simulink model "MdXX_RspOutComm"  (R2018b)
settings: Solver=FixedStepDiscrete  StartTime=0.0  StopTime=10.0  FixedStep=0.01  RelTol=1e-3
undefined symbols (not defined in the file or in its folder): KeSMSuRspStatHldTm_Val
libraries: RspLib x60
(part 1 of 2)
settings Model: Creator=sn2xws  LastModifiedBy=sn2xws
settings DataIOCC: SaveFormat=StructureWithTime
settings OptimizationCC: DefaultParameterBehavior=Inlined  EnhancedBackFolding=on  PassReuseOutputArgsAs=Individual arguments  ZeroExternalMemoryAtStartup=off  ZeroInternalMemoryAtStartup=off  OptimizeBlockOrder=speed  DifferentSizesBufferReuse=on  OptimizationCustomize=off
settings DebuggingCC: ParameterTunabilityLossMsg=error
settings ModelReferenceCC: ModelReferenceNumInstancesAllowed=Single
settings SFSimCC: MATLABDynamicMemAlloc=off
settings RTWCC: SystemTargetFile=autosar.tlc  GenCodeOnly=on  TemplateMakefile=ert_default_tmf  Description=AUTOSAR  GenerateReport=on  IncludeHyperlinkInReport=on  LaunchReport=on  GenerateTraceInfo=on  GenerateTraceReport=on  GenerateTraceReportSl=on  GenerateTraceReportSf=on  GenerateTraceReportEml=on
settings CodeAppCC: ForceParamTrailComments=on  IgnoreCustomStorageClasses=off  OperatorAnnotations=on  SimulinkDataObjDesc=on  SFDataObjDesc=on  InsertBlockDesc=on
settings STFCustomTargetCC: TargetLangStandard=C99 (ISO)  MultiwordLength=256  ParMdlRefBuildCompliant=on  CompOptLevelCompliant=on  IncludeMdlTerminateFcn=off  CombineOutputUpdateFcns=on  SuppressErrorStatus=on  ERTCustomFileBanners=on  SupportNonFinite=off  SupportComplex=off  SupportContinuousTime=off  SupportNonInlinedSFcns=off  RemoveResetFunc=on  MATLABClassNameForMDSCustomization=Simulink.SoftwareTarget.ERTCustomization  AutosarCompliant=on  UseToolchainInfoCompliant=on  LookupTableObjectStructAxisOrder=2,1,3,4,...  LUTObjectStructOrderEvenSpacing=Size,Table,Breakpoints  SystemTargetFile=autosar.tlc
settings ERTTargetCC: TargetLangStandard=C99 (ISO)  ConcurrentExecutionCompliant=off  IncludeMdlTerminateFcn=off  SuppressErrorStatus=on  SupportNonFinite=off  SupportComplex=off  ModelStepFunctionPrototypeControlCompliant=off  CPPClassGenCompliant=off  AutosarCompliant=on  LookupTableObjectStructAxisOrder=2,1,3,4,...  LUTObjectStructOrderEvenSpacing=Size,Table,Breakpoints  InlinedParameterPlacement=NonHierarchical  ERTCustomFileTemplate=example_file_process.tlc

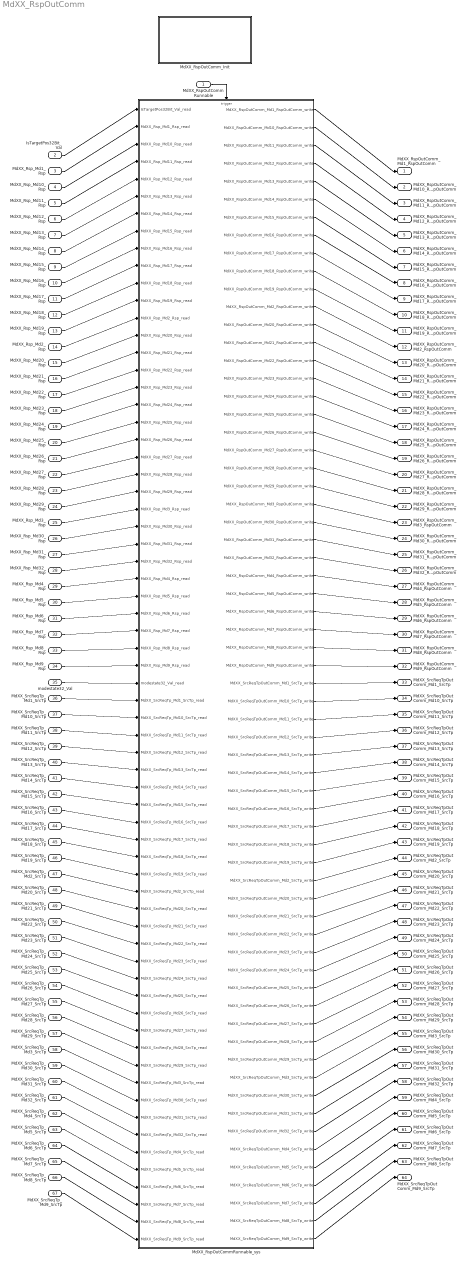
== system MdXX_RspOutComm ==
  MdXX_RspOutCommRunnable : Inport  SampleTime=0.01  OutputFunctionCall=on
  IsTargetPos32Bit_Val : Inport  Port=2  OutDataTypeStr=uint32  PortDimensions=1
  MdXX_Rsp_Md1_Rsp : Inport  Port=3  OutDataTypeStr=Enum: MdRspLocal2  PortDimensions=1
  MdXX_Rsp_Md10_Rsp : Inport  Port=4  OutDataTypeStr=Enum: MdRspLocal2  PortDimensions=1
  MdXX_Rsp_Md11_Rsp : Inport  Port=5  OutDataTypeStr=Enum: MdRspLocal2  PortDimensions=1
  MdXX_Rsp_Md12_Rsp : Inport  Port=6  OutDataTypeStr=Enum: MdRspLocal2  PortDimensions=1
  MdXX_Rsp_Md13_Rsp : Inport  Port=7  OutDataTypeStr=Enum: MdRspLocal2  PortDimensions=1
  MdXX_Rsp_Md14_Rsp : Inport  Port=8  OutDataTypeStr=Enum: MdRspLocal2  PortDimensions=1
  MdXX_Rsp_Md15_Rsp : Inport  Port=9  OutDataTypeStr=Enum: MdRspLocal2  PortDimensions=1
  MdXX_Rsp_Md16_Rsp : Inport  Port=10  OutDataTypeStr=Enum: MdRspLocal2  PortDimensions=1
  MdXX_Rsp_Md17_Rsp : Inport  Port=11  OutDataTypeStr=Enum: MdRspLocal2  PortDimensions=1
  MdXX_Rsp_Md18_Rsp : Inport  Port=12  OutDataTypeStr=Enum: MdRspLocal2  PortDimensions=1
  MdXX_Rsp_Md19_Rsp : Inport  Port=13  OutDataTypeStr=Enum: MdRspLocal2  PortDimensions=1
  MdXX_Rsp_Md2_Rsp : Inport  Port=14  OutDataTypeStr=Enum: MdRspLocal2  PortDimensions=1
  MdXX_Rsp_Md20_Rsp : Inport  Port=15  OutDataTypeStr=Enum: MdRspLocal2  PortDimensions=1
  MdXX_Rsp_Md21_Rsp : Inport  Port=16  OutDataTypeStr=Enum: MdRspLocal2  PortDimensions=1
  MdXX_Rsp_Md22_Rsp : Inport  Port=17  OutDataTypeStr=Enum: MdRspLocal2  PortDimensions=1
  MdXX_Rsp_Md23_Rsp : Inport  Port=18  OutDataTypeStr=Enum: MdRspLocal2  PortDimensions=1
  MdXX_Rsp_Md24_Rsp : Inport  Port=19  OutDataTypeStr=Enum: MdRspLocal2  PortDimensions=1
  MdXX_Rsp_Md25_Rsp : Inport  Port=20  OutDataTypeStr=Enum: MdRspLocal2  PortDimensions=1
  MdXX_Rsp_Md26_Rsp : Inport  Port=21  OutDataTypeStr=Enum: MdRspLocal2  PortDimensions=1
  MdXX_Rsp_Md27_Rsp : Inport  Port=22  OutDataTypeStr=Enum: MdRspLocal2  PortDimensions=1
  MdXX_Rsp_Md28_Rsp : Inport  Port=23  OutDataTypeStr=Enum: MdRspLocal2  PortDimensions=1
  MdXX_Rsp_Md29_Rsp : Inport  Port=24  OutDataTypeStr=Enum: MdRspLocal2  PortDimensions=1
  MdXX_Rsp_Md3_Rsp : Inport  Port=25  OutDataTypeStr=Enum: MdRspLocal2  PortDimensions=1
  MdXX_Rsp_Md30_Rsp : Inport  Port=26  OutDataTypeStr=Enum: MdRspLocal2  PortDimensions=1
  MdXX_Rsp_Md31_Rsp : Inport  Port=27  OutDataTypeStr=Enum: MdRspLocal2  PortDimensions=1
  MdXX_Rsp_Md32_Rsp : Inport  Port=28  OutDataTypeStr=Enum: MdRspLocal2  PortDimensions=1
  MdXX_Rsp_Md4_Rsp : Inport  Port=29  OutDataTypeStr=Enum: MdRspLocal2  PortDimensions=1
  MdXX_Rsp_Md5_Rsp : Inport  Port=30  OutDataTypeStr=Enum: MdRspLocal2  PortDimensions=1
  MdXX_Rsp_Md6_Rsp : Inport  Port=31  OutDataTypeStr=Enum: MdRspLocal2  PortDimensions=1
  MdXX_Rsp_Md7_Rsp : Inport  Port=32  OutDataTypeStr=Enum: MdRspLocal2  PortDimensions=1
  MdXX_Rsp_Md8_Rsp : Inport  Port=33  OutDataTypeStr=Enum: MdRspLocal2  PortDimensions=1
  MdXX_Rsp_Md9_Rsp : Inport  Port=34  OutDataTypeStr=Enum: MdRspLocal2  PortDimensions=1
  modestate32_Val : Inport  Port=35  OutDataTypeStr=uint32  PortDimensions=1
  MdXX_SrcReqTp_Md1_SrcTp : Inport  Port=36  OutDataTypeStr=Enum: SrcReqTp1  PortDimensions=1
  MdXX_SrcReqTp_Md10_SrcTp : Inport  Port=37  OutDataTypeStr=Enum: SrcReqTp1  PortDimensions=1
  MdXX_SrcReqTp_Md11_SrcTp : Inport  Port=38  OutDataTypeStr=Enum: SrcReqTp1  PortDimensions=1
  MdXX_SrcReqTp_Md12_SrcTp : Inport  Port=39  OutDataTypeStr=Enum: SrcReqTp1  PortDimensions=1
  MdXX_SrcReqTp_Md13_SrcTp : Inport  Port=40  OutDataTypeStr=Enum: SrcReqTp1  PortDimensions=1
  MdXX_SrcReqTp_Md14_SrcTp : Inport  Port=41  OutDataTypeStr=Enum: SrcReqTp1  PortDimensions=1
  MdXX_SrcReqTp_Md15_SrcTp : Inport  Port=42  OutDataTypeStr=Enum: SrcReqTp1  PortDimensions=1
  MdXX_SrcReqTp_Md16_SrcTp : Inport  Port=43  OutDataTypeStr=Enum: SrcReqTp1  PortDimensions=1
  MdXX_SrcReqTp_Md17_SrcTp : Inport  Port=44  OutDataTypeStr=Enum: SrcReqTp1  PortDimensions=1
  MdXX_SrcReqTp_Md18_SrcTp : Inport  Port=45  OutDataTypeStr=Enum: SrcReqTp1  PortDimensions=1
  MdXX_SrcReqTp_Md19_SrcTp : Inport  Port=46  OutDataTypeStr=Enum: SrcReqTp1  PortDimensions=1
  MdXX_SrcReqTp_Md2_SrcTp : Inport  Port=47  OutDataTypeStr=Enum: SrcReqTp1  PortDimensions=1
  MdXX_SrcReqTp_Md20_SrcTp : Inport  Port=48  OutDataTypeStr=Enum: SrcReqTp1  PortDimensions=1
  MdXX_SrcReqTp_Md21_SrcTp : Inport  Port=49  OutDataTypeStr=Enum: SrcReqTp1  PortDimensions=1
  MdXX_SrcReqTp_Md22_SrcTp : Inport  Port=50  OutDataTypeStr=Enum: SrcReqTp1  PortDimensions=1
  MdXX_SrcReqTp_Md23_SrcTp : Inport  Port=51  OutDataTypeStr=Enum: SrcReqTp1  PortDimensions=1
  MdXX_SrcReqTp_Md24_SrcTp : Inport  Port=52  OutDataTypeStr=Enum: SrcReqTp1  PortDimensions=1
  MdXX_SrcReqTp_Md25_SrcTp : Inport  Port=53  OutDataTypeStr=Enum: SrcReqTp1  PortDimensions=1
  MdXX_SrcReqTp_Md26_SrcTp : Inport  Port=54  OutDataTypeStr=Enum: SrcReqTp1  PortDimensions=1
  MdXX_SrcReqTp_Md27_SrcTp : Inport  Port=55  OutDataTypeStr=Enum: SrcReqTp1  PortDimensions=1
  MdXX_SrcReqTp_Md28_SrcTp : Inport  Port=56  OutDataTypeStr=Enum: SrcReqTp1  PortDimensions=1
  MdXX_SrcReqTp_Md29_SrcTp : Inport  Port=57  OutDataTypeStr=Enum: SrcReqTp1  PortDimensions=1
  MdXX_SrcReqTp_Md3_SrcTp : Inport  Port=58  OutDataTypeStr=Enum: SrcReqTp1  PortDimensions=1
  MdXX_SrcReqTp_Md30_SrcTp : Inport  Port=59  OutDataTypeStr=Enum: SrcReqTp1  PortDimensions=1
  MdXX_SrcReqTp_Md31_SrcTp : Inport  Port=60  OutDataTypeStr=Enum: SrcReqTp1  PortDimensions=1
  MdXX_SrcReqTp_Md32_SrcTp : Inport  Port=61  OutDataTypeStr=Enum: SrcReqTp1  PortDimensions=1
  MdXX_SrcReqTp_Md4_SrcTp : Inport  Port=62  OutDataTypeStr=Enum: SrcReqTp1  PortDimensions=1
  MdXX_SrcReqTp_Md5_SrcTp : Inport  Port=63  OutDataTypeStr=Enum: SrcReqTp1  PortDimensions=1
  MdXX_SrcReqTp_Md6_SrcTp : Inport  Port=64  OutDataTypeStr=Enum: SrcReqTp1  PortDimensions=1
  MdXX_SrcReqTp_Md7_SrcTp : Inport  Port=65  OutDataTypeStr=Enum: SrcReqTp1  PortDimensions=1
  MdXX_SrcReqTp_Md8_SrcTp : Inport  Port=66  OutDataTypeStr=Enum: SrcReqTp1  PortDimensions=1
  MdXX_SrcReqTp_Md9_SrcTp : Inport  Port=67  OutDataTypeStr=Enum: SrcReqTp1  PortDimensions=1
  MdXX_RspOutCommRunnable_sys : Subsystem
  MdXX_RspOutComm_Init : Subsystem
  MdXX_RspOutComm_Md1_RspOutComm : Outport  OutDataTypeStr=uint8  PortDimensions=1
  MdXX_RspOutComm_Md10_RspOutComm : Outport  Port=2  OutDataTypeStr=uint8  PortDimensions=1
  MdXX_RspOutComm_Md11_RspOutComm : Outport  Port=3  OutDataTypeStr=uint8  PortDimensions=1
  MdXX_RspOutComm_Md12_RspOutComm : Outport  Port=4  OutDataTypeStr=uint8  PortDimensions=1
  MdXX_RspOutComm_Md13_RspOutComm : Outport  Port=5  OutDataTypeStr=uint8  PortDimensions=1
  MdXX_RspOutComm_Md14_RspOutComm : Outport  Port=6  OutDataTypeStr=uint8  PortDimensions=1
  MdXX_RspOutComm_Md15_RspOutComm : Outport  Port=7  OutDataTypeStr=uint8  PortDimensions=1
  MdXX_RspOutComm_Md16_RspOutComm : Outport  Port=8  OutDataTypeStr=uint8  PortDimensions=1
  MdXX_RspOutComm_Md17_RspOutComm : Outport  Port=9  OutDataTypeStr=uint8  PortDimensions=1
  MdXX_RspOutComm_Md18_RspOutComm : Outport  Port=10  OutDataTypeStr=uint8  PortDimensions=1
  MdXX_RspOutComm_Md19_RspOutComm : Outport  Port=11  OutDataTypeStr=uint8  PortDimensions=1
  MdXX_RspOutComm_Md2_RspOutComm : Outport  Port=12  OutDataTypeStr=uint8  PortDimensions=1
  MdXX_RspOutComm_Md20_RspOutComm : Outport  Port=13  OutDataTypeStr=uint8  PortDimensions=1
  MdXX_RspOutComm_Md21_RspOutComm : Outport  Port=14  OutDataTypeStr=uint8  PortDimensions=1
  MdXX_RspOutComm_Md22_RspOutComm : Outport  Port=15  OutDataTypeStr=uint8  PortDimensions=1
  MdXX_RspOutComm_Md23_RspOutComm : Outport  Port=16  OutDataTypeStr=uint8  PortDimensions=1
  MdXX_RspOutComm_Md24_RspOutComm : Outport  Port=17  OutDataTypeStr=uint8  PortDimensions=1
  MdXX_RspOutComm_Md25_RspOutComm : Outport  Port=18  OutDataTypeStr=uint8  PortDimensions=1
  MdXX_RspOutComm_Md26_RspOutComm : Outport  Port=19  OutDataTypeStr=uint8  PortDimensions=1
  MdXX_RspOutComm_Md27_RspOutComm : Outport  Port=20  OutDataTypeStr=uint8  PortDimensions=1
  MdXX_RspOutComm_Md28_RspOutComm : Outport  Port=21  OutDataTypeStr=uint8  PortDimensions=1
  MdXX_RspOutComm_Md29_RspOutComm : Outport  Port=22  OutDataTypeStr=uint8  PortDimensions=1
  MdXX_RspOutComm_Md3_RspOutComm : Outport  Port=23  OutDataTypeStr=uint8  PortDimensions=1
  MdXX_RspOutComm_Md30_RspOutComm : Outport  Port=24  OutDataTypeStr=uint8  PortDimensions=1
  MdXX_RspOutComm_Md31_RspOutComm : Outport  Port=25  OutDataTypeStr=uint8  PortDimensions=1
  MdXX_RspOutComm_Md32_RspOutComm : Outport  Port=26  OutDataTypeStr=uint8  PortDimensions=1
  MdXX_RspOutComm_Md4_RspOutComm : Outport  Port=27  OutDataTypeStr=uint8  PortDimensions=1
  MdXX_RspOutComm_Md5_RspOutComm : Outport  Port=28  OutDataTypeStr=uint8  PortDimensions=1
  MdXX_RspOutComm_Md6_RspOutComm : Outport  Port=29  OutDataTypeStr=uint8  PortDimensions=1
  MdXX_RspOutComm_Md7_RspOutComm : Outport  Port=30  OutDataTypeStr=uint8  PortDimensions=1
  MdXX_RspOutComm_Md8_RspOutComm : Outport  Port=31  OutDataTypeStr=uint8  PortDimensions=1
  MdXX_RspOutComm_Md9_RspOutComm : Outport  Port=32  OutDataTypeStr=uint8  PortDimensions=1
  MdXX_SrcReqTpOutComm_Md1_SrcTp : Outport  Port=33  OutDataTypeStr=Enum: SrcReqTp1  PortDimensions=1
  MdXX_SrcReqTpOutComm_Md10_SrcTp : Outport  Port=34  OutDataTypeStr=Enum: SrcReqTp1  PortDimensions=1
  MdXX_SrcReqTpOutComm_Md11_SrcTp : Outport  Port=35  OutDataTypeStr=Enum: SrcReqTp1  PortDimensions=1
  MdXX_SrcReqTpOutComm_Md12_SrcTp : Outport  Port=36  OutDataTypeStr=Enum: SrcReqTp1  PortDimensions=1
  MdXX_SrcReqTpOutComm_Md13_SrcTp : Outport  Port=37  OutDataTypeStr=Enum: SrcReqTp1  PortDimensions=1
  MdXX_SrcReqTpOutComm_Md14_SrcTp : Outport  Port=38  OutDataTypeStr=Enum: SrcReqTp1  PortDimensions=1
  MdXX_SrcReqTpOutComm_Md15_SrcTp : Outport  Port=39  OutDataTypeStr=Enum: SrcReqTp1  PortDimensions=1
  MdXX_SrcReqTpOutComm_Md16_SrcTp : Outport  Port=40  OutDataTypeStr=Enum: SrcReqTp1  PortDimensions=1
  MdXX_SrcReqTpOutComm_Md17_SrcTp : Outport  Port=41  OutDataTypeStr=Enum: SrcReqTp1  PortDimensions=1
  MdXX_SrcReqTpOutComm_Md18_SrcTp : Outport  Port=42  OutDataTypeStr=Enum: SrcReqTp1  PortDimensions=1
  MdXX_SrcReqTpOutComm_Md19_SrcTp : Outport  Port=43  OutDataTypeStr=Enum: SrcReqTp1  PortDimensions=1
  MdXX_SrcReqTpOutComm_Md2_SrcTp : Outport  Port=44  OutDataTypeStr=Enum: SrcReqTp1  PortDimensions=1
  MdXX_SrcReqTpOutComm_Md20_SrcTp : Outport  Port=45  OutDataTypeStr=Enum: SrcReqTp1  PortDimensions=1
  MdXX_SrcReqTpOutComm_Md21_SrcTp : Outport  Port=46  OutDataTypeStr=Enum: SrcReqTp1  PortDimensions=1
  MdXX_SrcReqTpOutComm_Md22_SrcTp : Outport  Port=47  OutDataTypeStr=Enum: SrcReqTp1  PortDimensions=1
  MdXX_SrcReqTpOutComm_Md23_SrcTp : Outport  Port=48  OutDataTypeStr=Enum: SrcReqTp1  PortDimensions=1
  MdXX_SrcReqTpOutComm_Md24_SrcTp : Outport  Port=49  OutDataTypeStr=Enum: SrcReqTp1  PortDimensions=1
  MdXX_SrcReqTpOutComm_Md25_SrcTp : Outport  Port=50  OutDataTypeStr=Enum: SrcReqTp1  PortDimensions=1
  MdXX_SrcReqTpOutComm_Md26_SrcTp : Outport  Port=51  OutDataTypeStr=Enum: SrcReqTp1  PortDimensions=1
  MdXX_SrcReqTpOutComm_Md27_SrcTp : Outport  Port=52  OutDataTypeStr=Enum: SrcReqTp1  PortDimensions=1
  MdXX_SrcReqTpOutComm_Md28_SrcTp : Outport  Port=53  OutDataTypeStr=Enum: SrcReqTp1  PortDimensions=1
  MdXX_SrcReqTpOutComm_Md29_SrcTp : Outport  Port=54  OutDataTypeStr=Enum: SrcReqTp1  PortDimensions=1
  MdXX_SrcReqTpOutComm_Md3_SrcTp : Outport  Port=55  OutDataTypeStr=Enum: SrcReqTp1  PortDimensions=1
  MdXX_SrcReqTpOutComm_Md30_SrcTp : Outport  Port=56  OutDataTypeStr=Enum: SrcReqTp1  PortDimensions=1
  MdXX_SrcReqTpOutComm_Md31_SrcTp : Outport  Port=57  OutDataTypeStr=Enum: SrcReqTp1  PortDimensions=1
  MdXX_SrcReqTpOutComm_Md32_SrcTp : Outport  Port=58  OutDataTypeStr=Enum: SrcReqTp1  PortDimensions=1
  MdXX_SrcReqTpOutComm_Md4_SrcTp : Outport  Port=59  OutDataTypeStr=Enum: SrcReqTp1  PortDimensions=1
  MdXX_SrcReqTpOutComm_Md5_SrcTp : Outport  Port=60  OutDataTypeStr=Enum: SrcReqTp1  PortDimensions=1
  MdXX_SrcReqTpOutComm_Md6_SrcTp : Outport  Port=61  OutDataTypeStr=Enum: SrcReqTp1  PortDimensions=1
  MdXX_SrcReqTpOutComm_Md7_SrcTp : Outport  Port=62  OutDataTypeStr=Enum: SrcReqTp1  PortDimensions=1
  MdXX_SrcReqTpOutComm_Md8_SrcTp : Outport  Port=63  OutDataTypeStr=Enum: SrcReqTp1  PortDimensions=1
  MdXX_SrcReqTpOutComm_Md9_SrcTp : Outport  Port=64  OutDataTypeStr=Enum: SrcReqTp1  PortDimensions=1
  wires:
  IsTargetPos32Bit_Val/1 -> MdXX_RspOutCommRunnable_sys/1(IsTargetPos32Bit_Val_read)
  MdXX_Rsp_Md1_Rsp/1 -> MdXX_RspOutCommRunnable_sys/2(MdXX_Rsp_Md1_Rsp_read)
  MdXX_Rsp_Md10_Rsp/1 -> MdXX_RspOutCommRunnable_sys/3(MdXX_Rsp_Md10_Rsp_read)
  MdXX_Rsp_Md11_Rsp/1 -> MdXX_RspOutCommRunnable_sys/4(MdXX_Rsp_Md11_Rsp_read)
  MdXX_Rsp_Md12_Rsp/1 -> MdXX_RspOutCommRunnable_sys/5(MdXX_Rsp_Md12_Rsp_read)
  MdXX_Rsp_Md13_Rsp/1 -> MdXX_RspOutCommRunnable_sys/6(MdXX_Rsp_Md13_Rsp_read)
  MdXX_Rsp_Md14_Rsp/1 -> MdXX_RspOutCommRunnable_sys/7(MdXX_Rsp_Md14_Rsp_read)
  MdXX_Rsp_Md15_Rsp/1 -> MdXX_RspOutCommRunnable_sys/8(MdXX_Rsp_Md15_Rsp_read)
  MdXX_Rsp_Md16_Rsp/1 -> MdXX_RspOutCommRunnable_sys/9(MdXX_Rsp_Md16_Rsp_read)
  MdXX_Rsp_Md17_Rsp/1 -> MdXX_RspOutCommRunnable_sys/10(MdXX_Rsp_Md17_Rsp_read)
  MdXX_Rsp_Md18_Rsp/1 -> MdXX_RspOutCommRunnable_sys/11(MdXX_Rsp_Md18_Rsp_read)
  MdXX_Rsp_Md19_Rsp/1 -> MdXX_RspOutCommRunnable_sys/12(MdXX_Rsp_Md19_Rsp_read)
  MdXX_Rsp_Md2_Rsp/1 -> MdXX_RspOutCommRunnable_sys/13(MdXX_Rsp_Md2_Rsp_read)
  MdXX_Rsp_Md20_Rsp/1 -> MdXX_RspOutCommRunnable_sys/14(MdXX_Rsp_Md20_Rsp_read)
  MdXX_Rsp_Md21_Rsp/1 -> MdXX_RspOutCommRunnable_sys/15(MdXX_Rsp_Md21_Rsp_read)
  MdXX_Rsp_Md22_Rsp/1 -> MdXX_RspOutCommRunnable_sys/16(MdXX_Rsp_Md22_Rsp_read)
  MdXX_Rsp_Md23_Rsp/1 -> MdXX_RspOutCommRunnable_sys/17(MdXX_Rsp_Md23_Rsp_read)
  MdXX_Rsp_Md24_Rsp/1 -> MdXX_RspOutCommRunnable_sys/18(MdXX_Rsp_Md24_Rsp_read)
  MdXX_Rsp_Md25_Rsp/1 -> MdXX_RspOutCommRunnable_sys/19(MdXX_Rsp_Md25_Rsp_read)
  MdXX_Rsp_Md26_Rsp/1 -> MdXX_RspOutCommRunnable_sys/20(MdXX_Rsp_Md26_Rsp_read)
  MdXX_Rsp_Md27_Rsp/1 -> MdXX_RspOutCommRunnable_sys/21(MdXX_Rsp_Md27_Rsp_read)
  MdXX_Rsp_Md28_Rsp/1 -> MdXX_RspOutCommRunnable_sys/22(MdXX_Rsp_Md28_Rsp_read)
  MdXX_Rsp_Md29_Rsp/1 -> MdXX_RspOutCommRunnable_sys/23(MdXX_Rsp_Md29_Rsp_read)
  MdXX_Rsp_Md3_Rsp/1 -> MdXX_RspOutCommRunnable_sys/24(MdXX_Rsp_Md3_Rsp_read)
  MdXX_Rsp_Md30_Rsp/1 -> MdXX_RspOutCommRunnable_sys/25(MdXX_Rsp_Md30_Rsp_read)
  MdXX_Rsp_Md31_Rsp/1 -> MdXX_RspOutCommRunnable_sys/26(MdXX_Rsp_Md31_Rsp_read)
  MdXX_Rsp_Md32_Rsp/1 -> MdXX_RspOutCommRunnable_sys/27(MdXX_Rsp_Md32_Rsp_read)
  MdXX_Rsp_Md4_Rsp/1 -> MdXX_RspOutCommRunnable_sys/28(MdXX_Rsp_Md4_Rsp_read)
  MdXX_Rsp_Md5_Rsp/1 -> MdXX_RspOutCommRunnable_sys/29(MdXX_Rsp_Md5_Rsp_read)
  MdXX_Rsp_Md6_Rsp/1 -> MdXX_RspOutCommRunnable_sys/30(MdXX_Rsp_Md6_Rsp_read)
  MdXX_Rsp_Md7_Rsp/1 -> MdXX_RspOutCommRunnable_sys/31(MdXX_Rsp_Md7_Rsp_read)
  MdXX_Rsp_Md8_Rsp/1 -> MdXX_RspOutCommRunnable_sys/32(MdXX_Rsp_Md8_Rsp_read)
  MdXX_Rsp_Md9_Rsp/1 -> MdXX_RspOutCommRunnable_sys/33(MdXX_Rsp_Md9_Rsp_read)
  modestate32_Val/1 -> MdXX_RspOutCommRunnable_sys/34(modestate32_Val_read)
  MdXX_RspOutCommRunnable/1 -> MdXX_RspOutCommRunnable_sys/Trigger
  MdXX_RspOutCommRunnable_sys/1(MdXX_RspOutComm_Md1_RspOutComm_write) -> MdXX_RspOutComm_Md1_RspOutComm/1
  MdXX_RspOutCommRunnable_sys/2(MdXX_RspOutComm_Md10_RspOutComm_write) -> MdXX_RspOutComm_Md10_RspOutComm/1
  MdXX_RspOutCommRunnable_sys/3(MdXX_RspOutComm_Md11_RspOutComm_write) -> MdXX_RspOutComm_Md11_RspOutComm/1
  MdXX_RspOutCommRunnable_sys/4(MdXX_RspOutComm_Md12_RspOutComm_write) -> MdXX_RspOutComm_Md12_RspOutComm/1
  MdXX_RspOutCommRunnable_sys/5(MdXX_RspOutComm_Md13_RspOutComm_write) -> MdXX_RspOutComm_Md13_RspOutComm/1
  MdXX_RspOutCommRunnable_sys/6(MdXX_RspOutComm_Md14_RspOutComm_write) -> MdXX_RspOutComm_Md14_RspOutComm/1
  MdXX_RspOutCommRunnable_sys/7(MdXX_RspOutComm_Md15_RspOutComm_write) -> MdXX_RspOutComm_Md15_RspOutComm/1
  MdXX_RspOutCommRunnable_sys/8(MdXX_RspOutComm_Md16_RspOutComm_write) -> MdXX_RspOutComm_Md16_RspOutComm/1
  MdXX_RspOutCommRunnable_sys/9(MdXX_RspOutComm_Md17_RspOutComm_write) -> MdXX_RspOutComm_Md17_RspOutComm/1
  MdXX_RspOutCommRunnable_sys/10(MdXX_RspOutComm_Md18_RspOutComm_write) -> MdXX_RspOutComm_Md18_RspOutComm/1
  MdXX_RspOutCommRunnable_sys/11(MdXX_RspOutComm_Md19_RspOutComm_write) -> MdXX_RspOutComm_Md19_RspOutComm/1
  MdXX_RspOutCommRunnable_sys/12(MdXX_RspOutComm_Md2_RspOutComm_write) -> MdXX_RspOutComm_Md2_RspOutComm/1
  MdXX_RspOutCommRunnable_sys/13(MdXX_RspOutComm_Md20_RspOutComm_write) -> MdXX_RspOutComm_Md20_RspOutComm/1
  MdXX_RspOutCommRunnable_sys/14(MdXX_RspOutComm_Md21_RspOutComm_write) -> MdXX_RspOutComm_Md21_RspOutComm/1
  MdXX_RspOutCommRunnable_sys/15(MdXX_RspOutComm_Md22_RspOutComm_write) -> MdXX_RspOutComm_Md22_RspOutComm/1
  MdXX_RspOutCommRunnable_sys/16(MdXX_RspOutComm_Md23_RspOutComm_write) -> MdXX_RspOutComm_Md23_RspOutComm/1
  MdXX_RspOutCommRunnable_sys/17(MdXX_RspOutComm_Md24_RspOutComm_write) -> MdXX_RspOutComm_Md24_RspOutComm/1
  MdXX_RspOutCommRunnable_sys/18(MdXX_RspOutComm_Md25_RspOutComm_write) -> MdXX_RspOutComm_Md25_RspOutComm/1
  MdXX_RspOutCommRunnable_sys/19(MdXX_RspOutComm_Md26_RspOutComm_write) -> MdXX_RspOutComm_Md26_RspOutComm/1
  MdXX_RspOutCommRunnable_sys/20(MdXX_RspOutComm_Md27_RspOutComm_write) -> MdXX_RspOutComm_Md27_RspOutComm/1
  MdXX_RspOutCommRunnable_sys/21(MdXX_RspOutComm_Md28_RspOutComm_write) -> MdXX_RspOutComm_Md28_RspOutComm/1
  MdXX_RspOutCommRunnable_sys/22(MdXX_RspOutComm_Md29_RspOutComm_write) -> MdXX_RspOutComm_Md29_RspOutComm/1
  MdXX_RspOutCommRunnable_sys/23(MdXX_RspOutComm_Md3_RspOutComm_write) -> MdXX_RspOutComm_Md3_RspOutComm/1
  MdXX_RspOutCommRunnable_sys/24(MdXX_RspOutComm_Md30_RspOutComm_write) -> MdXX_RspOutComm_Md30_RspOutComm/1
  MdXX_RspOutCommRunnable_sys/25(MdXX_RspOutComm_Md31_RspOutComm_write) -> MdXX_RspOutComm_Md31_RspOutComm/1
  MdXX_RspOutCommRunnable_sys/26(MdXX_RspOutComm_Md32_RspOutComm_write) -> MdXX_RspOutComm_Md32_RspOutComm/1
  MdXX_RspOutCommRunnable_sys/27(MdXX_RspOutComm_Md4_RspOutComm_write) -> MdXX_RspOutComm_Md4_RspOutComm/1
  MdXX_RspOutCommRunnable_sys/28(MdXX_RspOutComm_Md5_RspOutComm_write) -> MdXX_RspOutComm_Md5_RspOutComm/1
  MdXX_RspOutCommRunnable_sys/29(MdXX_RspOutComm_Md6_RspOutComm_write) -> MdXX_RspOutComm_Md6_RspOutComm/1
  MdXX_RspOutCommRunnable_sys/30(MdXX_RspOutComm_Md7_RspOutComm_write) -> MdXX_RspOutComm_Md7_RspOutComm/1
  MdXX_RspOutCommRunnable_sys/31(MdXX_RspOutComm_Md8_RspOutComm_write) -> MdXX_RspOutComm_Md8_RspOutComm/1
  MdXX_RspOutCommRunnable_sys/32(MdXX_RspOutComm_Md9_RspOutComm_write) -> MdXX_RspOutComm_Md9_RspOutComm/1
  MdXX_SrcReqTp_Md1_SrcTp/1 -> MdXX_RspOutCommRunnable_sys/35(MdXX_SrcReqTp_Md1_SrcTp_read)
  MdXX_SrcReqTp_Md10_SrcTp/1 -> MdXX_RspOutCommRunnable_sys/36(MdXX_SrcReqTp_Md10_SrcTp_read)
  MdXX_SrcReqTp_Md11_SrcTp/1 -> MdXX_RspOutCommRunnable_sys/37(MdXX_SrcReqTp_Md11_SrcTp_read)
  MdXX_SrcReqTp_Md12_SrcTp/1 -> MdXX_RspOutCommRunnable_sys/38(MdXX_SrcReqTp_Md12_SrcTp_read)
  MdXX_SrcReqTp_Md13_SrcTp/1 -> MdXX_RspOutCommRunnable_sys/39(MdXX_SrcReqTp_Md13_SrcTp_read)
  MdXX_SrcReqTp_Md14_SrcTp/1 -> MdXX_RspOutCommRunnable_sys/40(MdXX_SrcReqTp_Md14_SrcTp_read)
  MdXX_SrcReqTp_Md15_SrcTp/1 -> MdXX_RspOutCommRunnable_sys/41(MdXX_SrcReqTp_Md15_SrcTp_read)
  MdXX_SrcReqTp_Md16_SrcTp/1 -> MdXX_RspOutCommRunnable_sys/42(MdXX_SrcReqTp_Md16_SrcTp_read)
  MdXX_SrcReqTp_Md17_SrcTp/1 -> MdXX_RspOutCommRunnable_sys/43(MdXX_SrcReqTp_Md17_SrcTp_read)
  MdXX_SrcReqTp_Md18_SrcTp/1 -> MdXX_RspOutCommRunnable_sys/44(MdXX_SrcReqTp_Md18_SrcTp_read)
  MdXX_SrcReqTp_Md19_SrcTp/1 -> MdXX_RspOutCommRunnable_sys/45(MdXX_SrcReqTp_Md19_SrcTp_read)
  MdXX_SrcReqTp_Md2_SrcTp/1 -> MdXX_RspOutCommRunnable_sys/46(MdXX_SrcReqTp_Md2_SrcTp_read)
  MdXX_SrcReqTp_Md20_SrcTp/1 -> MdXX_RspOutCommRunnable_sys/47(MdXX_SrcReqTp_Md20_SrcTp_read)
  MdXX_SrcReqTp_Md21_SrcTp/1 -> MdXX_RspOutCommRunnable_sys/48(MdXX_SrcReqTp_Md21_SrcTp_read)
  MdXX_SrcReqTp_Md22_SrcTp/1 -> MdXX_RspOutCommRunnable_sys/49(MdXX_SrcReqTp_Md22_SrcTp_read)
  MdXX_SrcReqTp_Md23_SrcTp/1 -> MdXX_RspOutCommRunnable_sys/50(MdXX_SrcReqTp_Md23_SrcTp_read)
  MdXX_SrcReqTp_Md24_SrcTp/1 -> MdXX_RspOutCommRunnable_sys/51(MdXX_SrcReqTp_Md24_SrcTp_read)
  MdXX_SrcReqTp_Md25_SrcTp/1 -> MdXX_RspOutCommRunnable_sys/52(MdXX_SrcReqTp_Md25_SrcTp_read)
  MdXX_SrcReqTp_Md26_SrcTp/1 -> MdXX_RspOutCommRunnable_sys/53(MdXX_SrcReqTp_Md26_SrcTp_read)
  MdXX_SrcReqTp_Md27_SrcTp/1 -> MdXX_RspOutCommRunnable_sys/54(MdXX_SrcReqTp_Md27_SrcTp_read)
  MdXX_SrcReqTp_Md28_SrcTp/1 -> MdXX_RspOutCommRunnable_sys/55(MdXX_SrcReqTp_Md28_SrcTp_read)
  MdXX_SrcReqTp_Md29_SrcTp/1 -> MdXX_RspOutCommRunnable_sys/56(MdXX_SrcReqTp_Md29_SrcTp_read)
  MdXX_SrcReqTp_Md3_SrcTp/1 -> MdXX_RspOutCommRunnable_sys/57(MdXX_SrcReqTp_Md3_SrcTp_read)
  MdXX_SrcReqTp_Md30_SrcTp/1 -> MdXX_RspOutCommRunnable_sys/58(MdXX_SrcReqTp_Md30_SrcTp_read)
  MdXX_SrcReqTp_Md31_SrcTp/1 -> MdXX_RspOutCommRunnable_sys/59(MdXX_SrcReqTp_Md31_SrcTp_read)
  MdXX_SrcReqTp_Md32_SrcTp/1 -> MdXX_RspOutCommRunnable_sys/60(MdXX_SrcReqTp_Md32_SrcTp_read)
  MdXX_SrcReqTp_Md4_SrcTp/1 -> MdXX_RspOutCommRunnable_sys/61(MdXX_SrcReqTp_Md4_SrcTp_read)
  MdXX_SrcReqTp_Md5_SrcTp/1 -> MdXX_RspOutCommRunnable_sys/62(MdXX_SrcReqTp_Md5_SrcTp_read)
  MdXX_SrcReqTp_Md6_SrcTp/1 -> MdXX_RspOutCommRunnable_sys/63(MdXX_SrcReqTp_Md6_SrcTp_read)
  MdXX_SrcReqTp_Md7_SrcTp/1 -> MdXX_RspOutCommRunnable_sys/64(MdXX_SrcReqTp_Md7_SrcTp_read)
  MdXX_SrcReqTp_Md8_SrcTp/1 -> MdXX_RspOutCommRunnable_sys/65(MdXX_SrcReqTp_Md8_SrcTp_read)
  MdXX_SrcReqTp_Md9_SrcTp/1 -> MdXX_RspOutCommRunnable_sys/66(MdXX_SrcReqTp_Md9_SrcTp_read)
  MdXX_RspOutCommRunnable_sys/33(MdXX_SrcReqTpOutComm_Md1_SrcTp_write) -> MdXX_SrcReqTpOutComm_Md1_SrcTp/1
  MdXX_RspOutCommRunnable_sys/34(MdXX_SrcReqTpOutComm_Md10_SrcTp_write) -> MdXX_SrcReqTpOutComm_Md10_SrcTp/1
  MdXX_RspOutCommRunnable_sys/35(MdXX_SrcReqTpOutComm_Md11_SrcTp_write) -> MdXX_SrcReqTpOutComm_Md11_SrcTp/1
  MdXX_RspOutCommRunnable_sys/36(MdXX_SrcReqTpOutComm_Md12_SrcTp_write) -> MdXX_SrcReqTpOutComm_Md12_SrcTp/1
  MdXX_RspOutCommRunnable_sys/37(MdXX_SrcReqTpOutComm_Md13_SrcTp_write) -> MdXX_SrcReqTpOutComm_Md13_SrcTp/1
  MdXX_RspOutCommRunnable_sys/38(MdXX_SrcReqTpOutComm_Md14_SrcTp_write) -> MdXX_SrcReqTpOutComm_Md14_SrcTp/1
  MdXX_RspOutCommRunnable_sys/39(MdXX_SrcReqTpOutComm_Md15_SrcTp_write) -> MdXX_SrcReqTpOutComm_Md15_SrcTp/1
  MdXX_RspOutCommRunnable_sys/40(MdXX_SrcReqTpOutComm_Md16_SrcTp_write) -> MdXX_SrcReqTpOutComm_Md16_SrcTp/1
  MdXX_RspOutCommRunnable_sys/41(MdXX_SrcReqTpOutComm_Md17_SrcTp_write) -> MdXX_SrcReqTpOutComm_Md17_SrcTp/1
  MdXX_RspOutCommRunnable_sys/42(MdXX_SrcReqTpOutComm_Md18_SrcTp_write) -> MdXX_SrcReqTpOutComm_Md18_SrcTp/1
  MdXX_RspOutCommRunnable_sys/43(MdXX_SrcReqTpOutComm_Md19_SrcTp_write) -> MdXX_SrcReqTpOutComm_Md19_SrcTp/1
  MdXX_RspOutCommRunnable_sys/44(MdXX_SrcReqTpOutComm_Md2_SrcTp_write) -> MdXX_SrcReqTpOutComm_Md2_SrcTp/1
  MdXX_RspOutCommRunnable_sys/45(MdXX_SrcReqTpOutComm_Md20_SrcTp_write) -> MdXX_SrcReqTpOutComm_Md20_SrcTp/1
  MdXX_RspOutCommRunnable_sys/46(MdXX_SrcReqTpOutComm_Md21_SrcTp_write) -> MdXX_SrcReqTpOutComm_Md21_SrcTp/1
  MdXX_RspOutCommRunnable_sys/47(MdXX_SrcReqTpOutComm_Md22_SrcTp_write) -> MdXX_SrcReqTpOutComm_Md22_SrcTp/1
  MdXX_RspOutCommRunnable_sys/48(MdXX_SrcReqTpOutComm_Md23_SrcTp_write) -> MdXX_SrcReqTpOutComm_Md23_SrcTp/1
  MdXX_RspOutCommRunnable_sys/49(MdXX_SrcReqTpOutComm_Md24_SrcTp_write) -> MdXX_SrcReqTpOutComm_Md24_SrcTp/1
  MdXX_RspOutCommRunnable_sys/50(MdXX_SrcReqTpOutComm_Md25_SrcTp_write) -> MdXX_SrcReqTpOutComm_Md25_SrcTp/1
  MdXX_RspOutCommRunnable_sys/51(MdXX_SrcReqTpOutComm_Md26_SrcTp_write) -> MdXX_SrcReqTpOutComm_Md26_SrcTp/1
  MdXX_RspOutCommRunnable_sys/52(MdXX_SrcReqTpOutComm_Md27_SrcTp_write) -> MdXX_SrcReqTpOutComm_Md27_SrcTp/1
  MdXX_RspOutCommRunnable_sys/53(MdXX_SrcReqTpOutComm_Md28_SrcTp_write) -> MdXX_SrcReqTpOutComm_Md28_SrcTp/1
  MdXX_RspOutCommRunnable_sys/54(MdXX_SrcReqTpOutComm_Md29_SrcTp_write) -> MdXX_SrcReqTpOutComm_Md29_SrcTp/1
  MdXX_RspOutCommRunnable_sys/55(MdXX_SrcReqTpOutComm_Md3_SrcTp_write) -> MdXX_SrcReqTpOutComm_Md3_SrcTp/1
  MdXX_RspOutCommRunnable_sys/56(MdXX_SrcReqTpOutComm_Md30_SrcTp_write) -> MdXX_SrcReqTpOutComm_Md30_SrcTp/1
  MdXX_RspOutCommRunnable_sys/57(MdXX_SrcReqTpOutComm_Md31_SrcTp_write) -> MdXX_SrcReqTpOutComm_Md31_SrcTp/1
  MdXX_RspOutCommRunnable_sys/58(MdXX_SrcReqTpOutComm_Md32_SrcTp_write) -> MdXX_SrcReqTpOutComm_Md32_SrcTp/1
  MdXX_RspOutCommRunnable_sys/59(MdXX_SrcReqTpOutComm_Md4_SrcTp_write) -> MdXX_SrcReqTpOutComm_Md4_SrcTp/1
  MdXX_RspOutCommRunnable_sys/60(MdXX_SrcReqTpOutComm_Md5_SrcTp_write) -> MdXX_SrcReqTpOutComm_Md5_SrcTp/1
  MdXX_RspOutCommRunnable_sys/61(MdXX_SrcReqTpOutComm_Md6_SrcTp_write) -> MdXX_SrcReqTpOutComm_Md6_SrcTp/1
  MdXX_RspOutCommRunnable_sys/62(MdXX_SrcReqTpOutComm_Md7_SrcTp_write) -> MdXX_SrcReqTpOutComm_Md7_SrcTp/1
  MdXX_RspOutCommRunnable_sys/63(MdXX_SrcReqTpOutComm_Md8_SrcTp_write) -> MdXX_SrcReqTpOutComm_Md8_SrcTp/1
  MdXX_RspOutCommRunnable_sys/64(MdXX_SrcReqTpOutComm_Md9_SrcTp_write) -> MdXX_SrcReqTpOutComm_Md9_SrcTp/1

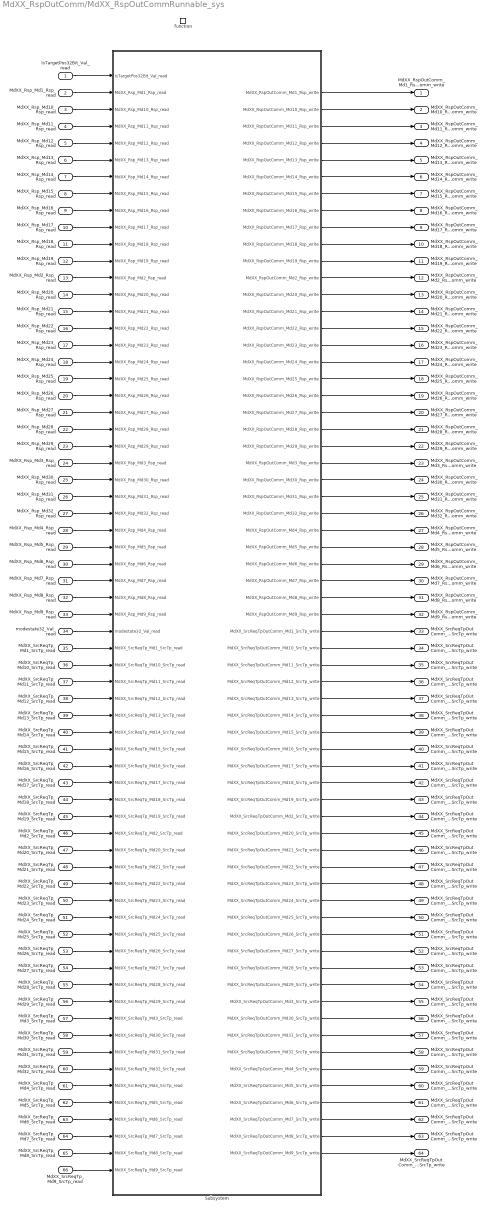
== system MdXX_RspOutComm/MdXX_RspOutCommRunnable_sys ==
  IsTargetPos32Bit_Val_read : Inport
  MdXX_Rsp_Md1_Rsp_read : Inport  Port=2
  MdXX_Rsp_Md10_Rsp_read : Inport  Port=3
  MdXX_Rsp_Md11_Rsp_read : Inport  Port=4
  MdXX_Rsp_Md12_Rsp_read : Inport  Port=5
  MdXX_Rsp_Md13_Rsp_read : Inport  Port=6
  MdXX_Rsp_Md14_Rsp_read : Inport  Port=7
  MdXX_Rsp_Md15_Rsp_read : Inport  Port=8
  MdXX_Rsp_Md16_Rsp_read : Inport  Port=9
  MdXX_Rsp_Md17_Rsp_read : Inport  Port=10
  MdXX_Rsp_Md18_Rsp_read : Inport  Port=11
  MdXX_Rsp_Md19_Rsp_read : Inport  Port=12
  MdXX_Rsp_Md2_Rsp_read : Inport  Port=13
  MdXX_Rsp_Md20_Rsp_read : Inport  Port=14
  MdXX_Rsp_Md21_Rsp_read : Inport  Port=15
  MdXX_Rsp_Md22_Rsp_read : Inport  Port=16
  MdXX_Rsp_Md23_Rsp_read : Inport  Port=17
  MdXX_Rsp_Md24_Rsp_read : Inport  Port=18
  MdXX_Rsp_Md25_Rsp_read : Inport  Port=19
  MdXX_Rsp_Md26_Rsp_read : Inport  Port=20
  MdXX_Rsp_Md27_Rsp_read : Inport  Port=21
  MdXX_Rsp_Md28_Rsp_read : Inport  Port=22
  MdXX_Rsp_Md29_Rsp_read : Inport  Port=23
  MdXX_Rsp_Md3_Rsp_read : Inport  Port=24
  MdXX_Rsp_Md30_Rsp_read : Inport  Port=25
  MdXX_Rsp_Md31_Rsp_read : Inport  Port=26
  MdXX_Rsp_Md32_Rsp_read : Inport  Port=27
  MdXX_Rsp_Md4_Rsp_read : Inport  Port=28
  MdXX_Rsp_Md5_Rsp_read : Inport  Port=29
  MdXX_Rsp_Md6_Rsp_read : Inport  Port=30
  MdXX_Rsp_Md7_Rsp_read : Inport  Port=31
  MdXX_Rsp_Md8_Rsp_read : Inport  Port=32
  MdXX_Rsp_Md9_Rsp_read : Inport  Port=33
  modestate32_Val_read : Inport  Port=34
  MdXX_SrcReqTp_Md1_SrcTp_read : Inport  Port=35
  MdXX_SrcReqTp_Md10_SrcTp_read : Inport  Port=36
  MdXX_SrcReqTp_Md11_SrcTp_read : Inport  Port=37
  MdXX_SrcReqTp_Md12_SrcTp_read : Inport  Port=38
  MdXX_SrcReqTp_Md13_SrcTp_read : Inport  Port=39
  MdXX_SrcReqTp_Md14_SrcTp_read : Inport  Port=40
  MdXX_SrcReqTp_Md15_SrcTp_read : Inport  Port=41
  MdXX_SrcReqTp_Md16_SrcTp_read : Inport  Port=42
  MdXX_SrcReqTp_Md17_SrcTp_read : Inport  Port=43
  MdXX_SrcReqTp_Md18_SrcTp_read : Inport  Port=44
  MdXX_SrcReqTp_Md19_SrcTp_read : Inport  Port=45
  MdXX_SrcReqTp_Md2_SrcTp_read : Inport  Port=46
  MdXX_SrcReqTp_Md20_SrcTp_read : Inport  Port=47
  MdXX_SrcReqTp_Md21_SrcTp_read : Inport  Port=48
  MdXX_SrcReqTp_Md22_SrcTp_read : Inport  Port=49
  MdXX_SrcReqTp_Md23_SrcTp_read : Inport  Port=50
  MdXX_SrcReqTp_Md24_SrcTp_read : Inport  Port=51
  MdXX_SrcReqTp_Md25_SrcTp_read : Inport  Port=52
  MdXX_SrcReqTp_Md26_SrcTp_read : Inport  Port=53
  MdXX_SrcReqTp_Md27_SrcTp_read : Inport  Port=54
  MdXX_SrcReqTp_Md28_SrcTp_read : Inport  Port=55
  MdXX_SrcReqTp_Md29_SrcTp_read : Inport  Port=56
  MdXX_SrcReqTp_Md3_SrcTp_read : Inport  Port=57
  MdXX_SrcReqTp_Md30_SrcTp_read : Inport  Port=58
  MdXX_SrcReqTp_Md31_SrcTp_read : Inport  Port=59
  MdXX_SrcReqTp_Md32_SrcTp_read : Inport  Port=60
  MdXX_SrcReqTp_Md4_SrcTp_read : Inport  Port=61
  MdXX_SrcReqTp_Md5_SrcTp_read : Inport  Port=62
  MdXX_SrcReqTp_Md6_SrcTp_read : Inport  Port=63
  MdXX_SrcReqTp_Md7_SrcTp_read : Inport  Port=64
  MdXX_SrcReqTp_Md8_SrcTp_read : Inport  Port=65
  MdXX_SrcReqTp_Md9_SrcTp_read : Inport  Port=66
  function : TriggerPort  TriggerType=function-call  VariantControl=(inherit)  SampleTimeType=periodic  SampleTime=-1
  Subsystem : Subsystem
  MdXX_RspOutComm_Md1_RspOutComm_write : Outport
      settings: EnsureOutportIsVirtual=on
  MdXX_RspOutComm_Md10_RspOutComm_write : Outport  Port=2
      settings: EnsureOutportIsVirtual=on
  MdXX_RspOutComm_Md11_RspOutComm_write : Outport  Port=3
      settings: EnsureOutportIsVirtual=on
  MdXX_RspOutComm_Md12_RspOutComm_write : Outport  Port=4
      settings: EnsureOutportIsVirtual=on
  MdXX_RspOutComm_Md13_RspOutComm_write : Outport  Port=5
      settings: EnsureOutportIsVirtual=on
  MdXX_RspOutComm_Md14_RspOutComm_write : Outport  Port=6
      settings: EnsureOutportIsVirtual=on
  MdXX_RspOutComm_Md15_RspOutComm_write : Outport  Port=7
      settings: EnsureOutportIsVirtual=on
  MdXX_RspOutComm_Md16_RspOutComm_write : Outport  Port=8
      settings: EnsureOutportIsVirtual=on
  MdXX_RspOutComm_Md17_RspOutComm_write : Outport  Port=9
      settings: EnsureOutportIsVirtual=on
  MdXX_RspOutComm_Md18_RspOutComm_write : Outport  Port=10
      settings: EnsureOutportIsVirtual=on
  MdXX_RspOutComm_Md19_RspOutComm_write : Outport  Port=11
      settings: EnsureOutportIsVirtual=on
  MdXX_RspOutComm_Md2_RspOutComm_write : Outport  Port=12
      settings: EnsureOutportIsVirtual=on
  MdXX_RspOutComm_Md20_RspOutComm_write : Outport  Port=13
      settings: EnsureOutportIsVirtual=on
  MdXX_RspOutComm_Md21_RspOutComm_write : Outport  Port=14
      settings: EnsureOutportIsVirtual=on
  MdXX_RspOutComm_Md22_RspOutComm_write : Outport  Port=15
      settings: EnsureOutportIsVirtual=on
  MdXX_RspOutComm_Md23_RspOutComm_write : Outport  Port=16
      settings: EnsureOutportIsVirtual=on
  MdXX_RspOutComm_Md24_RspOutComm_write : Outport  Port=17
      settings: EnsureOutportIsVirtual=on
  MdXX_RspOutComm_Md25_RspOutComm_write : Outport  Port=18
      settings: EnsureOutportIsVirtual=on
  MdXX_RspOutComm_Md26_RspOutComm_write : Outport  Port=19
      settings: EnsureOutportIsVirtual=on
  MdXX_RspOutComm_Md27_RspOutComm_write : Outport  Port=20
      settings: EnsureOutportIsVirtual=on
  MdXX_RspOutComm_Md28_RspOutComm_write : Outport  Port=21
      settings: EnsureOutportIsVirtual=on
  MdXX_RspOutComm_Md29_RspOutComm_write : Outport  Port=22
      settings: EnsureOutportIsVirtual=on
  MdXX_RspOutComm_Md3_RspOutComm_write : Outport  Port=23
      settings: EnsureOutportIsVirtual=on
  MdXX_RspOutComm_Md30_RspOutComm_write : Outport  Port=24
      settings: EnsureOutportIsVirtual=on
  MdXX_RspOutComm_Md31_RspOutComm_write : Outport  Port=25
      settings: EnsureOutportIsVirtual=on
  MdXX_RspOutComm_Md32_RspOutComm_write : Outport  Port=26
      settings: EnsureOutportIsVirtual=on
  MdXX_RspOutComm_Md4_RspOutComm_write : Outport  Port=27
      settings: EnsureOutportIsVirtual=on
  MdXX_RspOutComm_Md5_RspOutComm_write : Outport  Port=28
      settings: EnsureOutportIsVirtual=on
  MdXX_RspOutComm_Md6_RspOutComm_write : Outport  Port=29
      settings: EnsureOutportIsVirtual=on
  MdXX_RspOutComm_Md7_RspOutComm_write : Outport  Port=30
      settings: EnsureOutportIsVirtual=on
  MdXX_RspOutComm_Md8_RspOutComm_write : Outport  Port=31
      settings: EnsureOutportIsVirtual=on
  MdXX_RspOutComm_Md9_RspOutComm_write : Outport  Port=32
      settings: EnsureOutportIsVirtual=on
  MdXX_SrcReqTpOutComm_Md1_SrcTp_write : Outport  Port=33
      settings: EnsureOutportIsVirtual=on
  MdXX_SrcReqTpOutComm_Md10_SrcTp_write : Outport  Port=34
      settings: EnsureOutportIsVirtual=on
  MdXX_SrcReqTpOutComm_Md11_SrcTp_write : Outport  Port=35
      settings: EnsureOutportIsVirtual=on
  MdXX_SrcReqTpOutComm_Md12_SrcTp_write : Outport  Port=36
      settings: EnsureOutportIsVirtual=on
  MdXX_SrcReqTpOutComm_Md13_SrcTp_write : Outport  Port=37
      settings: EnsureOutportIsVirtual=on
  MdXX_SrcReqTpOutComm_Md14_SrcTp_write : Outport  Port=38
      settings: EnsureOutportIsVirtual=on
  MdXX_SrcReqTpOutComm_Md15_SrcTp_write : Outport  Port=39
      settings: EnsureOutportIsVirtual=on
  MdXX_SrcReqTpOutComm_Md16_SrcTp_write : Outport  Port=40
      settings: EnsureOutportIsVirtual=on
  MdXX_SrcReqTpOutComm_Md17_SrcTp_write : Outport  Port=41
      settings: EnsureOutportIsVirtual=on
  MdXX_SrcReqTpOutComm_Md18_SrcTp_write : Outport  Port=42
      settings: EnsureOutportIsVirtual=on
  MdXX_SrcReqTpOutComm_Md19_SrcTp_write : Outport  Port=43
      settings: EnsureOutportIsVirtual=on
  MdXX_SrcReqTpOutComm_Md2_SrcTp_write : Outport  Port=44
      settings: EnsureOutportIsVirtual=on
  MdXX_SrcReqTpOutComm_Md20_SrcTp_write : Outport  Port=45
      settings: EnsureOutportIsVirtual=on
  MdXX_SrcReqTpOutComm_Md21_SrcTp_write : Outport  Port=46
      settings: EnsureOutportIsVirtual=on
  MdXX_SrcReqTpOutComm_Md22_SrcTp_write : Outport  Port=47
      settings: EnsureOutportIsVirtual=on
  MdXX_SrcReqTpOutComm_Md23_SrcTp_write : Outport  Port=48
      settings: EnsureOutportIsVirtual=on
  MdXX_SrcReqTpOutComm_Md24_SrcTp_write : Outport  Port=49
      settings: EnsureOutportIsVirtual=on
  MdXX_SrcReqTpOutComm_Md25_SrcTp_write : Outport  Port=50
      settings: EnsureOutportIsVirtual=on
  MdXX_SrcReqTpOutComm_Md26_SrcTp_write : Outport  Port=51
      settings: EnsureOutportIsVirtual=on
  MdXX_SrcReqTpOutComm_Md27_SrcTp_write : Outport  Port=52
      settings: EnsureOutportIsVirtual=on
  MdXX_SrcReqTpOutComm_Md28_SrcTp_write : Outport  Port=53
      settings: EnsureOutportIsVirtual=on
  MdXX_SrcReqTpOutComm_Md29_SrcTp_write : Outport  Port=54
      settings: EnsureOutportIsVirtual=on
  MdXX_SrcReqTpOutComm_Md3_SrcTp_write : Outport  Port=55
      settings: EnsureOutportIsVirtual=on
  MdXX_SrcReqTpOutComm_Md30_SrcTp_write : Outport  Port=56
      settings: EnsureOutportIsVirtual=on
  MdXX_SrcReqTpOutComm_Md31_SrcTp_write : Outport  Port=57
      settings: EnsureOutportIsVirtual=on
  MdXX_SrcReqTpOutComm_Md32_SrcTp_write : Outport  Port=58
      settings: EnsureOutportIsVirtual=on
  MdXX_SrcReqTpOutComm_Md4_SrcTp_write : Outport  Port=59
      settings: EnsureOutportIsVirtual=on
  MdXX_SrcReqTpOutComm_Md5_SrcTp_write : Outport  Port=60
      settings: EnsureOutportIsVirtual=on
  MdXX_SrcReqTpOutComm_Md6_SrcTp_write : Outport  Port=61
      settings: EnsureOutportIsVirtual=on
  MdXX_SrcReqTpOutComm_Md7_SrcTp_write : Outport  Port=62
      settings: EnsureOutportIsVirtual=on
  MdXX_SrcReqTpOutComm_Md8_SrcTp_write : Outport  Port=63
      settings: EnsureOutportIsVirtual=on
  MdXX_SrcReqTpOutComm_Md9_SrcTp_write : Outport  Port=64
      settings: EnsureOutportIsVirtual=on
  wires:
  IsTargetPos32Bit_Val_read/1 -> Subsystem/1(IsTargetPos32Bit_Val_read)
  MdXX_Rsp_Md1_Rsp_read/1 -> Subsystem/2(MdXX_Rsp_Md1_Rsp_read)
  MdXX_Rsp_Md10_Rsp_read/1 -> Subsystem/3(MdXX_Rsp_Md10_Rsp_read)
  MdXX_Rsp_Md11_Rsp_read/1 -> Subsystem/4(MdXX_Rsp_Md11_Rsp_read)
  MdXX_Rsp_Md12_Rsp_read/1 -> Subsystem/5(MdXX_Rsp_Md12_Rsp_read)
  MdXX_Rsp_Md13_Rsp_read/1 -> Subsystem/6(MdXX_Rsp_Md13_Rsp_read)
  MdXX_Rsp_Md14_Rsp_read/1 -> Subsystem/7(MdXX_Rsp_Md14_Rsp_read)
  MdXX_Rsp_Md15_Rsp_read/1 -> Subsystem/8(MdXX_Rsp_Md15_Rsp_read)
  MdXX_Rsp_Md16_Rsp_read/1 -> Subsystem/9(MdXX_Rsp_Md16_Rsp_read)
  MdXX_Rsp_Md17_Rsp_read/1 -> Subsystem/10(MdXX_Rsp_Md17_Rsp_read)
  MdXX_Rsp_Md18_Rsp_read/1 -> Subsystem/11(MdXX_Rsp_Md18_Rsp_read)
  MdXX_Rsp_Md19_Rsp_read/1 -> Subsystem/12(MdXX_Rsp_Md19_Rsp_read)
  MdXX_Rsp_Md2_Rsp_read/1 -> Subsystem/13(MdXX_Rsp_Md2_Rsp_read)
  MdXX_Rsp_Md20_Rsp_read/1 -> Subsystem/14(MdXX_Rsp_Md20_Rsp_read)
  MdXX_Rsp_Md21_Rsp_read/1 -> Subsystem/15(MdXX_Rsp_Md21_Rsp_read)
  MdXX_Rsp_Md22_Rsp_read/1 -> Subsystem/16(MdXX_Rsp_Md22_Rsp_read)
  MdXX_Rsp_Md23_Rsp_read/1 -> Subsystem/17(MdXX_Rsp_Md23_Rsp_read)
  MdXX_Rsp_Md24_Rsp_read/1 -> Subsystem/18(MdXX_Rsp_Md24_Rsp_read)
  MdXX_Rsp_Md25_Rsp_read/1 -> Subsystem/19(MdXX_Rsp_Md25_Rsp_read)
  MdXX_Rsp_Md26_Rsp_read/1 -> Subsystem/20(MdXX_Rsp_Md26_Rsp_read)
  MdXX_Rsp_Md27_Rsp_read/1 -> Subsystem/21(MdXX_Rsp_Md27_Rsp_read)
  MdXX_Rsp_Md28_Rsp_read/1 -> Subsystem/22(MdXX_Rsp_Md28_Rsp_read)
  MdXX_Rsp_Md29_Rsp_read/1 -> Subsystem/23(MdXX_Rsp_Md29_Rsp_read)
  MdXX_Rsp_Md3_Rsp_read/1 -> Subsystem/24(MdXX_Rsp_Md3_Rsp_read)
  MdXX_Rsp_Md30_Rsp_read/1 -> Subsystem/25(MdXX_Rsp_Md30_Rsp_read)
  MdXX_Rsp_Md31_Rsp_read/1 -> Subsystem/26(MdXX_Rsp_Md31_Rsp_read)
  MdXX_Rsp_Md32_Rsp_read/1 -> Subsystem/27(MdXX_Rsp_Md32_Rsp_read)
  MdXX_Rsp_Md4_Rsp_read/1 -> Subsystem/28(MdXX_Rsp_Md4_Rsp_read)
  MdXX_Rsp_Md5_Rsp_read/1 -> Subsystem/29(MdXX_Rsp_Md5_Rsp_read)
  MdXX_Rsp_Md6_Rsp_read/1 -> Subsystem/30(MdXX_Rsp_Md6_Rsp_read)
  MdXX_Rsp_Md7_Rsp_read/1 -> Subsystem/31(MdXX_Rsp_Md7_Rsp_read)
  MdXX_Rsp_Md8_Rsp_read/1 -> Subsystem/32(MdXX_Rsp_Md8_Rsp_read)
  MdXX_Rsp_Md9_Rsp_read/1 -> Subsystem/33(MdXX_Rsp_Md9_Rsp_read)
  modestate32_Val_read/1 -> Subsystem/34(modestate32_Val_read)
  Subsystem/1(MdXX_RspOutComm_Md1_Rsp_write) -> MdXX_RspOutComm_Md1_RspOutComm_write/1
  Subsystem/2(MdXX_RspOutComm_Md10_Rsp_write) -> MdXX_RspOutComm_Md10_RspOutComm_write/1
  Subsystem/3(MdXX_RspOutComm_Md11_Rsp_write) -> MdXX_RspOutComm_Md11_RspOutComm_write/1
  Subsystem/4(MdXX_RspOutComm_Md12_Rsp_write) -> MdXX_RspOutComm_Md12_RspOutComm_write/1
  Subsystem/5(MdXX_RspOutComm_Md13_Rsp_write) -> MdXX_RspOutComm_Md13_RspOutComm_write/1
  Subsystem/6(MdXX_RspOutComm_Md14_Rsp_write) -> MdXX_RspOutComm_Md14_RspOutComm_write/1
  Subsystem/7(MdXX_RspOutComm_Md15_Rsp_write) -> MdXX_RspOutComm_Md15_RspOutComm_write/1
  Subsystem/8(MdXX_RspOutComm_Md16_Rsp_write) -> MdXX_RspOutComm_Md16_RspOutComm_write/1
  Subsystem/9(MdXX_RspOutComm_Md17_Rsp_write) -> MdXX_RspOutComm_Md17_RspOutComm_write/1
  Subsystem/10(MdXX_RspOutComm_Md18_Rsp_write) -> MdXX_RspOutComm_Md18_RspOutComm_write/1
  Subsystem/11(MdXX_RspOutComm_Md19_Rsp_write) -> MdXX_RspOutComm_Md19_RspOutComm_write/1
  Subsystem/12(MdXX_RspOutComm_Md2_Rsp_write) -> MdXX_RspOutComm_Md2_RspOutComm_write/1
  Subsystem/13(MdXX_RspOutComm_Md20_Rsp_write) -> MdXX_RspOutComm_Md20_RspOutComm_write/1
  Subsystem/14(MdXX_RspOutComm_Md21_Rsp_write) -> MdXX_RspOutComm_Md21_RspOutComm_write/1
  Subsystem/15(MdXX_RspOutComm_Md22_Rsp_write) -> MdXX_RspOutComm_Md22_RspOutComm_write/1
  Subsystem/16(MdXX_RspOutComm_Md23_Rsp_write) -> MdXX_RspOutComm_Md23_RspOutComm_write/1
  Subsystem/17(MdXX_RspOutComm_Md24_Rsp_write) -> MdXX_RspOutComm_Md24_RspOutComm_write/1
  Subsystem/18(MdXX_RspOutComm_Md25_Rsp_write) -> MdXX_RspOutComm_Md25_RspOutComm_write/1
  Subsystem/19(MdXX_RspOutComm_Md26_Rsp_write) -> MdXX_RspOutComm_Md26_RspOutComm_write/1
  Subsystem/20(MdXX_RspOutComm_Md27_Rsp_write) -> MdXX_RspOutComm_Md27_RspOutComm_write/1
  Subsystem/21(MdXX_RspOutComm_Md28_Rsp_write) -> MdXX_RspOutComm_Md28_RspOutComm_write/1
  Subsystem/22(MdXX_RspOutComm_Md29_Rsp_write) -> MdXX_RspOutComm_Md29_RspOutComm_write/1
  Subsystem/23(MdXX_RspOutComm_Md3_Rsp_write) -> MdXX_RspOutComm_Md3_RspOutComm_write/1
  Subsystem/24(MdXX_RspOutComm_Md30_Rsp_write) -> MdXX_RspOutComm_Md30_RspOutComm_write/1
  Subsystem/25(MdXX_RspOutComm_Md31_Rsp_write) -> MdXX_RspOutComm_Md31_RspOutComm_write/1
  Subsystem/26(MdXX_RspOutComm_Md32_Rsp_write) -> MdXX_RspOutComm_Md32_RspOutComm_write/1
  Subsystem/27(MdXX_RspOutComm_Md4_Rsp_write) -> MdXX_RspOutComm_Md4_RspOutComm_write/1
  Subsystem/28(MdXX_RspOutComm_Md5_Rsp_write) -> MdXX_RspOutComm_Md5_RspOutComm_write/1
  Subsystem/29(MdXX_RspOutComm_Md6_Rsp_write) -> MdXX_RspOutComm_Md6_RspOutComm_write/1
  Subsystem/30(MdXX_RspOutComm_Md7_Rsp_write) -> MdXX_RspOutComm_Md7_RspOutComm_write/1
  Subsystem/31(MdXX_RspOutComm_Md8_Rsp_write) -> MdXX_RspOutComm_Md8_RspOutComm_write/1
  Subsystem/32(MdXX_RspOutComm_Md9_Rsp_write) -> MdXX_RspOutComm_Md9_RspOutComm_write/1
  MdXX_SrcReqTp_Md1_SrcTp_read/1 -> Subsystem/35(MdXX_SrcReqTp_Md1_SrcTp_read)
  MdXX_SrcReqTp_Md10_SrcTp_read/1 -> Subsystem/36(MdXX_SrcReqTp_Md10_SrcTp_read)
  MdXX_SrcReqTp_Md11_SrcTp_read/1 -> Subsystem/37(MdXX_SrcReqTp_Md11_SrcTp_read)
  MdXX_SrcReqTp_Md12_SrcTp_read/1 -> Subsystem/38(MdXX_SrcReqTp_Md12_SrcTp_read)
  MdXX_SrcReqTp_Md13_SrcTp_read/1 -> Subsystem/39(MdXX_SrcReqTp_Md13_SrcTp_read)
  MdXX_SrcReqTp_Md14_SrcTp_read/1 -> Subsystem/40(MdXX_SrcReqTp_Md14_SrcTp_read)
  MdXX_SrcReqTp_Md15_SrcTp_read/1 -> Subsystem/41(MdXX_SrcReqTp_Md15_SrcTp_read)
  MdXX_SrcReqTp_Md16_SrcTp_read/1 -> Subsystem/42(MdXX_SrcReqTp_Md16_SrcTp_read)
  MdXX_SrcReqTp_Md17_SrcTp_read/1 -> Subsystem/43(MdXX_SrcReqTp_Md17_SrcTp_read)
  MdXX_SrcReqTp_Md18_SrcTp_read/1 -> Subsystem/44(MdXX_SrcReqTp_Md18_SrcTp_read)
  MdXX_SrcReqTp_Md19_SrcTp_read/1 -> Subsystem/45(MdXX_SrcReqTp_Md19_SrcTp_read)
  MdXX_SrcReqTp_Md2_SrcTp_read/1 -> Subsystem/46(MdXX_SrcReqTp_Md2_SrcTp_read)
  MdXX_SrcReqTp_Md20_SrcTp_read/1 -> Subsystem/47(MdXX_SrcReqTp_Md20_SrcTp_read)
  MdXX_SrcReqTp_Md21_SrcTp_read/1 -> Subsystem/48(MdXX_SrcReqTp_Md21_SrcTp_read)
  MdXX_SrcReqTp_Md22_SrcTp_read/1 -> Subsystem/49(MdXX_SrcReqTp_Md22_SrcTp_read)
  MdXX_SrcReqTp_Md23_SrcTp_read/1 -> Subsystem/50(MdXX_SrcReqTp_Md23_SrcTp_read)
  MdXX_SrcReqTp_Md24_SrcTp_read/1 -> Subsystem/51(MdXX_SrcReqTp_Md24_SrcTp_read)
  MdXX_SrcReqTp_Md25_SrcTp_read/1 -> Subsystem/52(MdXX_SrcReqTp_Md25_SrcTp_read)
  MdXX_SrcReqTp_Md26_SrcTp_read/1 -> Subsystem/53(MdXX_SrcReqTp_Md26_SrcTp_read)
  MdXX_SrcReqTp_Md27_SrcTp_read/1 -> Subsystem/54(MdXX_SrcReqTp_Md27_SrcTp_read)
  MdXX_SrcReqTp_Md28_SrcTp_read/1 -> Subsystem/55(MdXX_SrcReqTp_Md28_SrcTp_read)
  MdXX_SrcReqTp_Md29_SrcTp_read/1 -> Subsystem/56(MdXX_SrcReqTp_Md29_SrcTp_read)
  MdXX_SrcReqTp_Md3_SrcTp_read/1 -> Subsystem/57(MdXX_SrcReqTp_Md3_SrcTp_read)
  MdXX_SrcReqTp_Md30_SrcTp_read/1 -> Subsystem/58(MdXX_SrcReqTp_Md30_SrcTp_read)
  MdXX_SrcReqTp_Md31_SrcTp_read/1 -> Subsystem/59(MdXX_SrcReqTp_Md31_SrcTp_read)
  MdXX_SrcReqTp_Md32_SrcTp_read/1 -> Subsystem/60(MdXX_SrcReqTp_Md32_SrcTp_read)
  MdXX_SrcReqTp_Md4_SrcTp_read/1 -> Subsystem/61(MdXX_SrcReqTp_Md4_SrcTp_read)
  MdXX_SrcReqTp_Md5_SrcTp_read/1 -> Subsystem/62(MdXX_SrcReqTp_Md5_SrcTp_read)
  MdXX_SrcReqTp_Md6_SrcTp_read/1 -> Subsystem/63(MdXX_SrcReqTp_Md6_SrcTp_read)
  MdXX_SrcReqTp_Md7_SrcTp_read/1 -> Subsystem/64(MdXX_SrcReqTp_Md7_SrcTp_read)
  MdXX_SrcReqTp_Md8_SrcTp_read/1 -> Subsystem/65(MdXX_SrcReqTp_Md8_SrcTp_read)
  MdXX_SrcReqTp_Md9_SrcTp_read/1 -> Subsystem/66(MdXX_SrcReqTp_Md9_SrcTp_read)
  Subsystem/33(MdXX_SrcReqTpOutComm_Md1_SrcTp_write) -> MdXX_SrcReqTpOutComm_Md1_SrcTp_write/1
  Subsystem/34(MdXX_SrcReqTpOutComm_Md10_SrcTp_write) -> MdXX_SrcReqTpOutComm_Md10_SrcTp_write/1
  Subsystem/35(MdXX_SrcReqTpOutComm_Md11_SrcTp_write) -> MdXX_SrcReqTpOutComm_Md11_SrcTp_write/1
  Subsystem/36(MdXX_SrcReqTpOutComm_Md12_SrcTp_write) -> MdXX_SrcReqTpOutComm_Md12_SrcTp_write/1
  Subsystem/37(MdXX_SrcReqTpOutComm_Md13_SrcTp_write) -> MdXX_SrcReqTpOutComm_Md13_SrcTp_write/1
  Subsystem/38(MdXX_SrcReqTpOutComm_Md14_SrcTp_write) -> MdXX_SrcReqTpOutComm_Md14_SrcTp_write/1
  Subsystem/39(MdXX_SrcReqTpOutComm_Md15_SrcTp_write) -> MdXX_SrcReqTpOutComm_Md15_SrcTp_write/1
  Subsystem/40(MdXX_SrcReqTpOutComm_Md16_SrcTp_write) -> MdXX_SrcReqTpOutComm_Md16_SrcTp_write/1
  Subsystem/41(MdXX_SrcReqTpOutComm_Md17_SrcTp_write) -> MdXX_SrcReqTpOutComm_Md17_SrcTp_write/1
  Subsystem/42(MdXX_SrcReqTpOutComm_Md18_SrcTp_write) -> MdXX_SrcReqTpOutComm_Md18_SrcTp_write/1
  Subsystem/43(MdXX_SrcReqTpOutComm_Md19_SrcTp_write) -> MdXX_SrcReqTpOutComm_Md19_SrcTp_write/1
  Subsystem/44(MdXX_SrcReqTpOutComm_Md2_SrcTp_write) -> MdXX_SrcReqTpOutComm_Md2_SrcTp_write/1
  Subsystem/45(MdXX_SrcReqTpOutComm_Md20_SrcTp_write) -> MdXX_SrcReqTpOutComm_Md20_SrcTp_write/1
  Subsystem/46(MdXX_SrcReqTpOutComm_Md21_SrcTp_write) -> MdXX_SrcReqTpOutComm_Md21_SrcTp_write/1
  Subsystem/47(MdXX_SrcReqTpOutComm_Md22_SrcTp_write) -> MdXX_SrcReqTpOutComm_Md22_SrcTp_write/1
  Subsystem/48(MdXX_SrcReqTpOutComm_Md23_SrcTp_write) -> MdXX_SrcReqTpOutComm_Md23_SrcTp_write/1
  Subsystem/49(MdXX_SrcReqTpOutComm_Md24_SrcTp_write) -> MdXX_SrcReqTpOutComm_Md24_SrcTp_write/1
  Subsystem/50(MdXX_SrcReqTpOutComm_Md25_SrcTp_write) -> MdXX_SrcReqTpOutComm_Md25_SrcTp_write/1
  Subsystem/51(MdXX_SrcReqTpOutComm_Md26_SrcTp_write) -> MdXX_SrcReqTpOutComm_Md26_SrcTp_write/1
  Subsystem/52(MdXX_SrcReqTpOutComm_Md27_SrcTp_write) -> MdXX_SrcReqTpOutComm_Md27_SrcTp_write/1
  Subsystem/53(MdXX_SrcReqTpOutComm_Md28_SrcTp_write) -> MdXX_SrcReqTpOutComm_Md28_SrcTp_write/1
  Subsystem/54(MdXX_SrcReqTpOutComm_Md29_SrcTp_write) -> MdXX_SrcReqTpOutComm_Md29_SrcTp_write/1
  Subsystem/55(MdXX_SrcReqTpOutComm_Md3_SrcTp_write) -> MdXX_SrcReqTpOutComm_Md3_SrcTp_write/1
  Subsystem/56(MdXX_SrcReqTpOutComm_Md30_SrcTp_write) -> MdXX_SrcReqTpOutComm_Md30_SrcTp_write/1
  Subsystem/57(MdXX_SrcReqTpOutComm_Md31_SrcTp_write) -> MdXX_SrcReqTpOutComm_Md31_SrcTp_write/1
  Subsystem/58(MdXX_SrcReqTpOutComm_Md32_SrcTp_write) -> MdXX_SrcReqTpOutComm_Md32_SrcTp_write/1
  Subsystem/59(MdXX_SrcReqTpOutComm_Md4_SrcTp_write) -> MdXX_SrcReqTpOutComm_Md4_SrcTp_write/1
  Subsystem/60(MdXX_SrcReqTpOutComm_Md5_SrcTp_write) -> MdXX_SrcReqTpOutComm_Md5_SrcTp_write/1
  Subsystem/61(MdXX_SrcReqTpOutComm_Md6_SrcTp_write) -> MdXX_SrcReqTpOutComm_Md6_SrcTp_write/1
  Subsystem/62(MdXX_SrcReqTpOutComm_Md7_SrcTp_write) -> MdXX_SrcReqTpOutComm_Md7_SrcTp_write/1
  Subsystem/63(MdXX_SrcReqTpOutComm_Md8_SrcTp_write) -> MdXX_SrcReqTpOutComm_Md8_SrcTp_write/1
  Subsystem/64(MdXX_SrcReqTpOutComm_Md9_SrcTp_write) -> MdXX_SrcReqTpOutComm_Md9_SrcTp_write/1

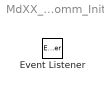
== system MdXX_RspOutComm/MdXX_RspOutComm_Init ==
  Event Listener : EventListener  EventName=reset
